simulink model "sim_BTMS"  (R2018b)
settings: Solver=FixedStepAuto  StartTime=0.0  StopTime=SimPara.t_sim  FixedStep=SimPara.t_step  RelTol=1e-3
values from neighbouring files (symbols this model uses):
  p = epe(jj).p    [main_sim_BTMS.m]    (also in main_sim_BTMS_1_system_setup.m = epe_mod(jj).p)
  SysPara = rmfield(SysPara, {'p','s'})    [main_sim_BTMS_1_system_setup.m]
undefined symbols (not defined in the file or in its folder): A, BatPara, BTMSConfig, i, LSAPara, SimPara, x2_cal, x3_cal, x_cal
libraries: simulink x14, dspstat3 x7, dspindex x1
(part 1 of 4)
Description:
  | A framework for the design and simulation of lithium-ion battery systems including the consideration of battery thermal management systems (BTMS).
  | Refer to https://github.com/TUMFTM/sim_BTMS for futher information.
  | 
  | Authors:
  | 
  | Christoph Reiter (christoph.reiter@tum.de)
  | Lars-Eric Schlereth
  | 
  | Created at:
  | 
  | Institute of Automotive Technology
  | Department of Mechanical Engineering
  | Technical University of Munich
settings Model: SimulationMode=accelerator  Creator=Christoph Reiter  LastModifiedBy=gu74niw
settings DataIOCC: SaveOutput=off  SignalLogging=off  DSMLogging=off  SaveTime=off  ReturnWorkspaceOutputs=on
settings OptimizationCC: SimCompilerOptimization=on

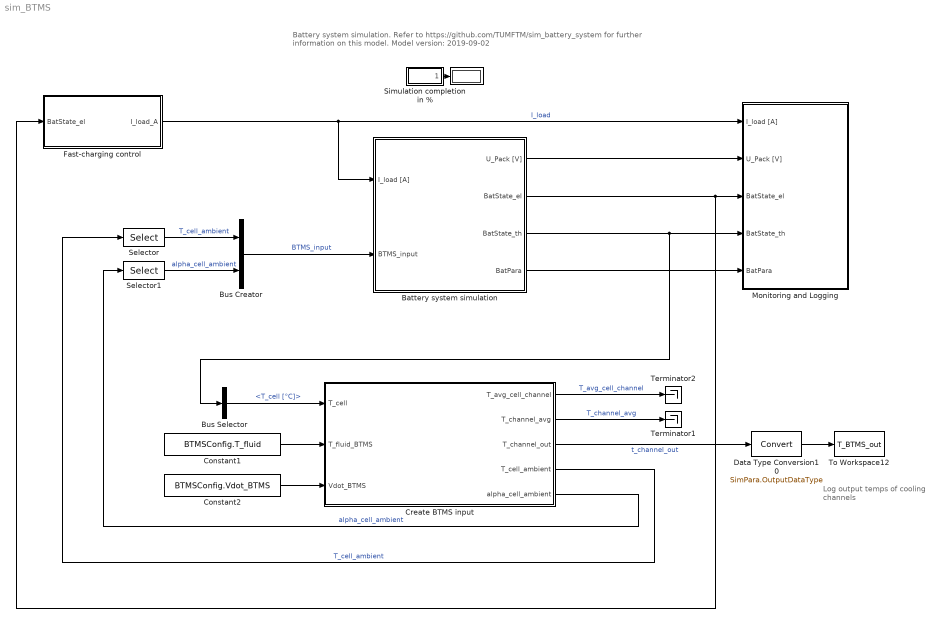
== system sim_BTMS ==
  note: Battery system simulation. Refer to https://github.com/TUMFTM/sim_battery_system for further information on this model.
      | Model version: 2019-09-02
  note: Log output temps of
      | cooling channels
  "\t\t      Simulation completion in %\t" : Subsystem
  " " : Display
      settings: Format=bank
  Battery system simulation : Subsystem  TreatAsAtomicUnit=on
  Bus Creator : BusCreator  Inputs=2
  Bus Selector : BusSelector  OutputSignals=T_cell [°C]
  Constant1 : Constant  Value=BTMSConfig.T_fluid
  Constant2 : Constant  Value=BTMSConfig.Vdot_BTMS
  Create BTMS input : Subsystem  Variant=on  VariantControl=Variant1
  Data Type Conversion10 : DataTypeConversion  OutDataTypeStr=SimPara.OutputDataType
  Fast-charging control : Subsystem
  Monitoring and Logging : Subsystem
  Selector : Selector  NumberOfDimensions=2  InputPortWidth=3  IndexOptions=Index vector (dialog),Index vector (dialog)  Indices=1:SysPara.p,1:SysPara.s  OutputSizes=1,1
  Selector1 : Selector  NumberOfDimensions=2  InputPortWidth=3  IndexOptions=Index vector (dialog),Index vector (dialog)  Indices=1:SysPara.p,1:SysPara.s  OutputSizes=1,1
  Terminator1 : Terminator
  Terminator2 : Terminator
  To Workspace12 : ToWorkspace  VariableName=T_BTMS_out  SaveFormat=Timeseries  SampleTime=-1
      settings: Decimation=SimPara.OutputDecimation
  wires:
  "\t\t      Simulation completion in %\t"/1(" ") -> " "/1
  Battery system simulation/1(U_Pack [V]) -> Monitoring and Logging/2(U_Pack [V])
  Battery system simulation/2(BatState_el) -> Fast-charging control/1(BatState_el), Monitoring and Logging/3(BatState_el)
  Battery system simulation/4(BatPara) -> Monitoring and Logging/5(BatPara)
  Battery system simulation/3(BatState_th) -> Bus Selector/1, Monitoring and Logging/4(BatState_th)
  Bus Creator/1 -> Battery system simulation/2(BTMS_input)  "BTMS_input"
  Bus Selector/1 -> Create BTMS input/1("T_cell ")  "<T_cell [°C]>"
  Constant1/1 -> Create BTMS input/2("T_fluid_BTMS ")
  Constant2/1 -> Create BTMS input/3("Vdot_BTMS ")
  Create BTMS input/1(" T_avg_cell_channel") -> Terminator2/1  "T_avg_cell_channel"
  Create BTMS input/3(" T_channel_out") -> Data Type Conversion10/1  "t_channel_out"
  Create BTMS input/4(" T_cell_ambient") -> Selector/1  "T_cell_ambient"
  Create BTMS input/5(" alpha_cell_ambient") -> Selector1/1  "alpha_cell_ambient"
  Create BTMS input/2(" T_channel_avg") -> Terminator1/1  "T_channel_avg"
  Fast-charging control/1(I_load_A) -> Battery system simulation/1(I_load [A]), Monitoring and Logging/1(I_load [A])  "I_load"
  Selector/1 -> Bus Creator/1  "T_cell_ambient"
  Selector1/1 -> Bus Creator/2  "alpha_cell_ambient"
  Data Type Conversion10/1 -> To Workspace12/1

== system sim_BTMS/		      Simulation completion in %	 ==
  note: Determine simulation completion
  Clock : Clock
  Divide : Product  Inputs=*/
  max. Simulaton Time : Constant  Value=SimPara.t_sim
  to % : Gain  Gain=100
  " " : Outport
  wires:
  max. Simulaton Time/1 -> Divide/2
  Clock/1 -> Divide/1
  Divide/1 -> to %/1
  to %/1 -> " "/1

== system sim_BTMS/Battery system simulation ==
  I_load [A] : Inport
  BTMS_input : Inport  Port=2
  Electrical Submodel : Subsystem
  Save BatState_el of last time-step : Subsystem
  Save BatState_th of last time-step : Subsystem
  Static and dynamic LIB parameters : Subsystem
  Thermal Submodel : Subsystem
  U_Pack [V] : Outport
  BatState_el : Outport  Port=2
  BatState_th : Outport  Port=3
  BatPara : Outport  Port=4
  wires:
  Static and dynamic LIB parameters/1(BatPara) -> Electrical Submodel/2(BatPara), Thermal Submodel/4(BatPara), BatPara/1
  Electrical Submodel/1(BatState_el) -> BatState_el/1, Save BatState_el of last time-step/1(BatState_el), Thermal Submodel/3(BatState_el)
  I_load [A]/1 -> Electrical Submodel/1(I_Pack [A])
  Electrical Submodel/2(U_Pack [V]) -> U_Pack [V]/1
  Save BatState_el of last time-step/1(BatState_el_in) -> Static and dynamic LIB parameters/2(BatState_el_in), Electrical Submodel/3(BatState_in)
  Thermal Submodel/1(BatState_th) -> BatState_th/1, Save BatState_th of last time-step/1(BatState_th)
  Save BatState_th of last time-step/1(Bat_State_th_in) -> Thermal Submodel/1(BatState_th_in), Static and dynamic LIB parameters/1(BatState_th_in)
  BTMS_input/1 -> Thermal Submodel/2(BTMS_input)

== system sim_BTMS/Create BTMS input ==
  "T_cell " : Inport
  "T_fluid_BTMS " : Inport  Port=2
  "Vdot_BTMS " : Inport  Port=3
  BTMS constant temp : Subsystem  VariantControl=SimPara.BTMS_sim_enable == 0
  BTMS fluid simulation : Subsystem  VariantControl=SimPara.BTMS_sim_enable == 1
  " T_avg_cell_channel" : Outport
  " T_channel_avg" : Outport  Port=2
  " T_channel_out" : Outport  Port=3
  " T_cell_ambient" : Outport  Port=4
  " alpha_cell_ambient" : Outport  Port=5

== system sim_BTMS/Fast-charging control ==
  note: Current reduction step
      | if max voltage is reached
  note: Detection of fully charged battery
  note: Overcharge-Protection
  BatState_el : Inport
  Add1 : Sum  Inputs=+-
  Battery fully charged : Constant  Value=SysPara.SOC_charge_max
  Bus Selector : BusSelector  OutputSignals=U_cell [V],SOC
  Constant1 : Constant  Value=SysPara.I_charge_min
  Constant2 : Constant
  Constant3 : Constant  Value=0
  Maximum : dspstat3/Maximum  operation=maximum  fcn=Value  indexBase=One  operateOver=Entire input  Dimension=1  InputProcessing=Columns as channels (frame based)  reset=None  roiEnable=off  roiType=Rectangles  roiPortion=Entire ROI  roiOutput=Individual statistics for each ROI  roiFlag=off  roundingMode=Floor  overflowMode=off  accumDataTypeStr=Inherit: Same as product output  accumLastDataTypeStr=Inherit: Same as product output
  Maximum1 : dspstat3/Maximum  operation=maximum  fcn=Value  indexBase=One  operateOver=Entire input  Dimension=1  InputProcessing=Columns as channels (frame based)  reset=None  roiEnable=off  roiType=Rectangles  roiPortion=Entire ROI  roiOutput=Individual statistics for each ROI  roiFlag=off  roundingMode=Floor  overflowMode=off  accumDataTypeStr=Inherit: Same as product output  accumLastDataTypeStr=Inherit: Same as product output
  Mean : dspstat3/Mean  run=off  InputProcessing=Columns as channels (frame based)  reset_popup=None  directionMode=Entire input  dimension=1  roiEnable=off  roiType=Rectangles  roiPortion=Entire ROI  roiOutput=Individual statistics for each ROI  roiFlag=off  roundingMode=Floor  overflowMode=off  outputDataTypeStr=Inherit: Same as accumulator  outputMin=[]  outputMax=[]  outputLastDataTypeStr=Inherit: Same as accumulator
  Relational Operator : RelationalOperator  OutDataTypeStr=boolean  RndMeth=Simplest
  Relational Operator2 : RelationalOperator  OutDataTypeStr=boolean  RndMeth=Simplest
  Stop Simulation : Stop
  Stop Simulation1 : Stop
  Switch1 : Switch  Threshold=SysPara.U_charge_target
  Unit Delay1 : UnitDelay  InitialCondition=SysPara.I_charge  SampleTime=-1
  Unit Delay2 : UnitDelay  InitialCondition=SysPara.I_charge  SampleTime=-1
  I_load_A : Outport
  wires:
  Unit Delay1/1 -> Add1/1
  Add1/1 -> Unit Delay1/1, Mean/1
  Relational Operator2/1 -> Stop Simulation1/1
  Switch1/1 -> Add1/2
  Constant1/1 -> Relational Operator2/1
  Constant2/1 -> Switch1/1
  Constant3/1 -> Switch1/3
  Bus Selector/1 -> Maximum/1  "<U_cell [V]>"
  Mean/1 -> Relational Operator2/2, Unit Delay2/1
  BatState_el/1 -> Bus Selector/1
  Maximum1/1 -> Relational Operator/1
  Battery fully charged/1 -> Relational Operator/2
  Relational Operator/1 -> Stop Simulation/1
  Bus Selector/2 -> Maximum1/1  "<SOC>"
  Maximum/1 -> Switch1/2
  Unit Delay2/1 -> I_load_A/1

== system sim_BTMS/Monitoring and Logging ==
  I_load [A] : Inport
  U_Pack [V] : Inport  Port=2
  BatState_el : Inport  Port=3
  BatState_th : Inport  Port=4
  BatPara : Inport  Port=5
  Constant : Constant  Value=SimPara.LoggingOutput
  Load Spectrum Analysis : Subsystem  Variant=on  VariantControl=Variant1
  Logging of Variables : Subsystem
  Temperature Sensor Simulation : Subsystem
  wires:
  I_load [A]/1 -> Logging of Variables/1(I_load [A])
  U_Pack [V]/1 -> Logging of Variables/2(U_Pack [A])
  BatState_el/1 -> Logging of Variables/3(BatState_el), Load Spectrum Analysis/1("BatState_el ")
  BatState_th/1 -> Temperature Sensor Simulation/1(bat_state_th_in)
  BatPara/1 -> Logging of Variables/5(BatPara), Load Spectrum Analysis/3("BatPara ")
  Constant/1 -> Logging of Variables/Enable
  Temperature Sensor Simulation/1(bat_state_th_out) -> Logging of Variables/4(BatState_th), Load Spectrum Analysis/2("BatState_th ")

== system sim_BTMS/Battery system simulation/Electrical Submodel ==
  note: Delay resulting balancing current for one step to avoid algebraic loop
  I_Pack [A] : Inport
  BatPara : Inport  Port=2
  BatState_in : Inport  Port=3
  Bus Creator1 : BusCreator  Inputs=8
  Cell Balancing : Subsystem
  Electric potential (single cell) : Subsystem
  Ohmic voltage drop and compensating currents in parallel connections : Subsystem
  Unit Delay4 : UnitDelay  InitialCondition=zeros(SysPara.p,SysPara.s)  SampleTime=-1
  Voltage of battery system : Subsystem
  dt : Subsystem
  BatState_el : Outport
  U_Pack [V] : Outport  Port=2
  wires:
  I_Pack [A]/1 -> Cell Balancing/1(I_Pack [A]), Ohmic voltage drop and compensating currents in parallel connections/2(I_Pack [A])
  Unit Delay4/1 -> Ohmic voltage drop and compensating currents in parallel connections/1(I_Balancing_in [A])  "I_Balancing_in [A]"
  Ohmic voltage drop and compensating currents in parallel connections/1(U_Cell [V]) -> Bus Creator1/1, Voltage of battery system/1(U_Cells [V]), Cell Balancing/2(U_Cell [V])
  Ohmic voltage drop and compensating currents in parallel connections/2(I_Cell [A]) -> Bus Creator1/2
  Ohmic voltage drop and compensating currents in parallel connections/3(U_R [V]) -> Bus Creator1/3
  Cell Balancing/1(I_Balancing [A]) -> Unit Delay4/1
  Voltage of battery system/1(U_Pack [V]) -> U_Pack [V]/1
  Bus Creator1/1 -> BatState_el/1  "BatState_el"
  BatPara/1 -> Ohmic voltage drop and compensating currents in parallel connections/3(BatPara), Electric potential (single cell)/1(BatPara)
  Electric potential (single cell)/1(U_Potential) -> Ohmic voltage drop and compensating currents in parallel connections/4(U_Potential [V]), Bus Creator1/4
  dt/1(dt [s]) -> Electric potential (single cell)/2(dt)
  BatState_in/1 -> Electric potential (single cell)/3(BatState_in)
  Electric potential (single cell)/2(SOC) -> Bus Creator1/5
  Electric potential (single cell)/3(U_OCV) -> Bus Creator1/6
  Electric potential (single cell)/4(U_Hysteresis) -> Bus Creator1/7
  Electric potential (single cell)/5(U_RC) -> Bus Creator1/8

== system sim_BTMS/Battery system simulation/Save BatState_el of last time-step ==
  note: Delay system state variables by one step to avoid algebraic loop.
      | We need these for the parameter lookup-tables
  BatState_el : Inport
  Bus Creator : BusCreator  Inputs=4
  Bus Creator2 : BusCreator  Inputs=4
  Bus Selector : BusSelector  OutputSignals=U_RC1 [V],U_RC2 [V],U_RC3 [V],U_RC4 [V]
  Bus Selector1 : BusSelector  OutputSignals=SOC,U_Hysteresis [V],I_cell [A],U_RC [V]
  Unit Delay : UnitDelay  InitialCondition=SysPara.BatStateInit.electrical.SOC  SampleTime=-1
  Unit Delay1 : UnitDelay  InitialCondition=SysPara.BatStateInit.electrical.U_hyst  SampleTime=-1
  Unit Delay2 : UnitDelay  InitialCondition=SysPara.BatStateInit.electrical.U_RC1  SampleTime=-1
  Unit Delay3 : UnitDelay  InitialCondition=SysPara.BatStateInit.electrical.U_RC2  SampleTime=-1
  Unit Delay4 : UnitDelay  InitialCondition=SysPara.BatStateInit.electrical.I_cell  SampleTime=-1
  Unit Delay5 : UnitDelay  InitialCondition=SysPara.BatStateInit.electrical.U_RC3  SampleTime=-1
  Unit Delay6 : UnitDelay  InitialCondition=SysPara.BatStateInit.electrical.U_RC4  SampleTime=-1
  BatState_el_in : Outport
  wires:
  Bus Selector1/2 -> Unit Delay1/1  "<U_Hysteresis [V]>"
  Unit Delay4/1 -> Bus Creator2/3  "I_cell [A]"
  Bus Selector1/3 -> Unit Delay4/1  "<I_cell [A]>"
  Unit Delay1/1 -> Bus Creator2/2  "U_Hysteresis [V]"
  Bus Selector1/1 -> Unit Delay/1  "<SOC>"
  Unit Delay/1 -> Bus Creator2/1  "SOC"
  Bus Creator2/1 -> BatState_el_in/1  "BatState_el_in"
  BatState_el/1 -> Bus Selector1/1
  Bus Selector1/4 -> Bus Selector/1  "<U_RC [V]>"
  Bus Selector/1 -> Unit Delay2/1  "<U_RC1 [V]>"
  Bus Selector/2 -> Unit Delay3/1  "<U_RC2 [V]>"
  Bus Selector/3 -> Unit Delay5/1  "<U_RC3 [V]>"
  Bus Selector/4 -> Unit Delay6/1  "<U_RC4 [V]>"
  Unit Delay6/1 -> Bus Creator/4  "U_RC4 [V]"
  Unit Delay5/1 -> Bus Creator/3  "U_RC3 [V]"
  Unit Delay3/1 -> Bus Creator/2  "U_RC2 [V]"
  Unit Delay2/1 -> Bus Creator/1  "U_RC1 [V]"
  Bus Creator/1 -> Bus Creator2/4  "U_RC"

== system sim_BTMS/Battery system simulation/Save BatState_th of last time-step ==
  note: Delay system state variables by one step to avoid algebraic loop.
      | We need these for the parameter lookup-tables
  BatState_th : Inport
  Bus Creator1 : BusCreator  Inputs=1
  Bus Selector : BusSelector  OutputSignals=T_cell [°C]
  Unit Delay1 : UnitDelay  InitialCondition=SysPara.BatStateInit.thermal.T_cell  SampleTime=-1
  Bat_State_th_in : Outport
  wires:
  Unit Delay1/1 -> Bus Creator1/1  "T_cell [°C]"
  Bus Selector/1 -> Unit Delay1/1  "<T_cell [°C]>"
  Bus Creator1/1 -> Bat_State_th_in/1  "Bat_State_th_in"
  BatState_th/1 -> Bus Selector/1

== system sim_BTMS/Battery system simulation/Static and dynamic LIB parameters ==
  BatState_th_in : Inport
  BatState_el_in : Inport  Port=2
  LIB Parameter Look-Ups : Subsystem
  Statistic Cell Deviations : Subsystem
  BatPara : Outport
  wires:
  LIB Parameter Look-Ups/1(BatPara_el_uniform) -> Statistic Cell Deviations/1("BatPara_el_uniform ")
  Statistic Cell Deviations/1(BatPara) -> BatPara/1  "BatPara"
  BatState_el_in/1 -> LIB Parameter Look-Ups/2(BatState_el_in)
  BatState_th_in/1 -> LIB Parameter Look-Ups/1(BatState_th_in)

== system sim_BTMS/Battery system simulation/Thermal Submodel ==
  note: Total cell heat generation:
      |
      | PQ_cell = PQ_cell,irr + PQ_cell,rev
  BatState_th_in : Inport
  BTMS_input : Inport  Port=2
  BatState_el : Inport  Port=3
  BatPara : Inport  Port=4
  Add : Sum
  Bus Creator : BusCreator  Inputs=6
  Bus Selector : BusSelector  OutputSignals=U_R [V],U_RC [V],I_cell [A]
  Bus Selector3 : BusSelector  OutputSignals=alpha_cell_ambient,T_cell_ambient
  Bus Selector4 : BusSelector  OutputSignals=T_cell [°C]
  Cell heat transport and heat dissipation : Subsystem
  Constant : Constant  Value=SimPara.thermal_sim_enable
  Irreversible heat generation : Subsystem
  Reversible heat generation : Subsystem
  BatState_th : Outport
  wires:
  Bus Selector3/2 -> Cell heat transport and heat dissipation/5(T_cell_ambient), Bus Creator/5  "<T_cell_ambient>"
  Add/1 -> Cell heat transport and heat dissipation/1(PQ_cell), Bus Creator/1  "PQ_cell [W]"
  Bus Creator/1 -> BatState_th/1  "BatState_th"
  Bus Selector3/1 -> Cell heat transport and heat dissipation/4(alpha_cell_ambient), Bus Creator/6  "<alpha_cell_ambient>"
  Irreversible heat generation/1(PQ_cell,irr [W]) -> Add/1
  Reversible heat generation/1(PQ_cell,rev [W]) -> Add/2
  BatPara/1 -> Cell heat transport and heat dissipation/2(BatPara), Reversible heat generation/3(BatPara)
  BatState_el/1 -> Bus Selector/1
  Bus Selector/2 -> Irreversible heat generation/2(U_RC)  "<U_RC [V]>"
  Bus Selector/3 -> Reversible heat generation/1(I_Cells [A]), Irreversible heat generation/3(I_Cells [A])  "<I_cell [A]>"
  Bus Selector/1 -> Irreversible heat generation/1(U_R [V])  "<U_R [V]>"
  BTMS_input/1 -> Bus Selector3/1
  BatState_th_in/1 -> Bus Selector4/1
  Bus Selector4/1 -> Reversible heat generation/2(T_Cells [°C]), Cell heat transport and heat dissipation/3(T_cell_in)  "<T_cell [°C]>"
  Cell heat transport and heat dissipation/1(T_cell [°C]) -> Bus Creator/2
  Constant/1 -> Cell heat transport and heat dissipation/Enable
  Cell heat transport and heat dissipation/3(PQ_transfer [W]) -> Bus Creator/4
  Cell heat transport and heat dissipation/2(PQ_ambient [W]) -> Bus Creator/3

== system sim_BTMS/Create BTMS input/BTMS constant temp ==
  note: BTMS simulation switched off, assuming constand ambient cell temperatures and heat transfer coefficients.
  "T_cell " : Inport
  "T_fluid_BTMS " : Inport  Port=2
  "Vdot_BTMS " : Inport  Port=3
  Constant : Constant  Value=SysPara.thermal.T_cell_ambient*ones(SysPara.p, SysPara.s)
  Constant3 : Constant  Value=SysPara.thermal.alpha_cell_ambient*ones(SysPara.p, SysPara.s)
  Ground : Ground
  Ground1 : Ground
  Ground2 : Ground
  Terminator : Terminator
  Terminator1 : Terminator
  Terminator2 : Terminator
  " T_avg_cell_channel" : Outport
  " T_channel_avg" : Outport  Port=2
  " T_channel_out" : Outport  Port=3
  " T_cell_ambient" : Outport  Port=4
  " alpha_cell_ambient" : Outport  Port=5
  wires:
  "T_cell "/1 -> Terminator/1
  "T_fluid_BTMS "/1 -> Terminator1/1
  "Vdot_BTMS "/1 -> Terminator2/1
  Ground1/1 -> " T_channel_avg"/1
  Constant/1 -> " T_cell_ambient"/1  "T_cell_ambient"
  Constant3/1 -> " alpha_cell_ambient"/1  "alpha_cell_ambient"
  Ground2/1 -> " T_channel_out"/1
  Ground/1 -> " T_avg_cell_channel"/1

== system sim_BTMS/Create BTMS input/BTMS fluid simulation ==
  note: Use T_cell of last time-step
      | to avoid algebraic loop
  "T_cell " : Inport
  "T_fluid_BTMS " : Inport  Port=2
  "Vdot_BTMS " : Inport  Port=3
  BTMS fluid simulation function : MATLAB Function  TreatAsAtomicUnit=on  VariantControl=Variant1
  Constant1 : Constant  Value=SysPara.thermal.transfer.A_y
  Constant2 : Constant  Value=SysPara.thermal.transfer.A_z
  Constant3 : Constant  Value=SysPara.thermal.transfer.A_x
  Constant4 : Constant  Value=SysPara.s
  Constant5 : Constant  Value=SysPara.p
  Unit Delay : UnitDelay  InitialCondition=SysPara.BatStateInit.electrical.SOC  SampleTime=-1
  " T_avg_cell_channel" : Outport
  " T_channel_avg" : Outport  Port=2
  " T_channel_out" : Outport  Port=3
  " T_cell_ambient" : Outport  Port=4
  " alpha_cell_ambient" : Outport  Port=5
  wires:
  "T_cell "/1 -> Unit Delay/1
  "T_fluid_BTMS "/1 -> BTMS fluid simulation function/2(T_fluid_BTMS)
  "Vdot_BTMS "/1 -> BTMS fluid simulation function/3(Vdot_BTMS)
  BTMS fluid simulation function/1(T_avg_cell_channel) -> " T_avg_cell_channel"/1
  BTMS fluid simulation function/2(T_channel_avg) -> " T_channel_avg"/1
  BTMS fluid simulation function/3(T_channel_out) -> " T_channel_out"/1
  BTMS fluid simulation function/4(T_cell_ambient) -> " T_cell_ambient"/1
  BTMS fluid simulation function/5(alpha_cell_ambient) -> " alpha_cell_ambient"/1
  Constant3/1 -> BTMS fluid simulation function/4(A_x)  "alpha_cell_ambient"
  Constant1/1 -> BTMS fluid simulation function/5(A_y)  "alpha_cell_ambient"
  Constant2/1 -> BTMS fluid simulation function/6(A_z)  "alpha_cell_ambient"
  Constant4/1 -> BTMS fluid simulation function/7(s)  "alpha_cell_ambient"
  Constant5/1 -> BTMS fluid simulation function/8(p)  "alpha_cell_ambient"
  Unit Delay/1 -> BTMS fluid simulation function/1(T_cell)  "T_cell"

== system sim_BTMS/Monitoring and Logging/Load Spectrum Analysis ==
  "BatState_el " : Inport
  "BatState_th " : Inport  Port=2
  "BatPara " : Inport  Port=3
  Load Spectrum Analysis OFF : Subsystem  VariantControl=SimPara.LoadSpectra_enable == 0
  Load Spectrum Analysis ON : Subsystem  VariantControl=SimPara.LoadSpectra_enable == 1

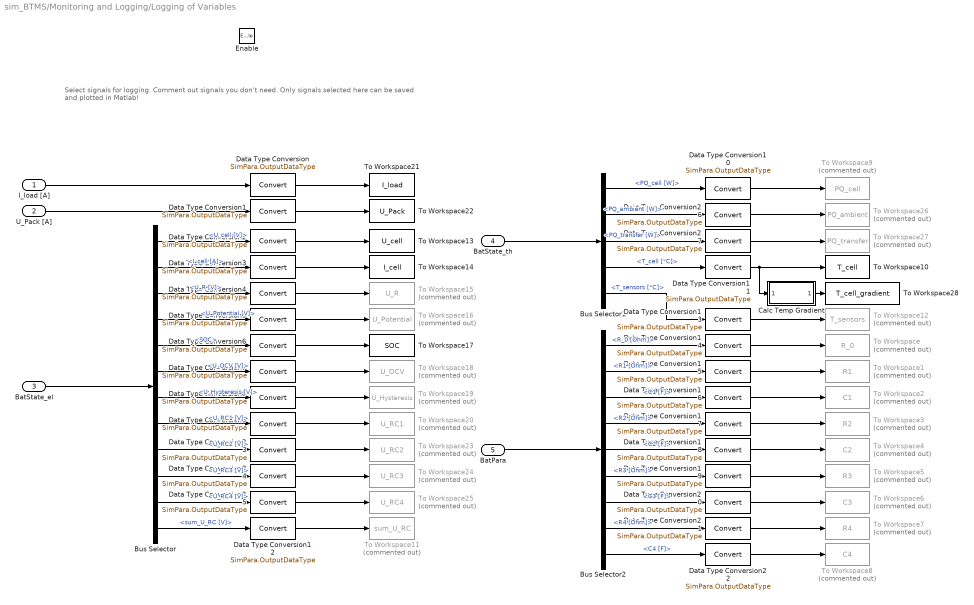
== system sim_BTMS/Monitoring and Logging/Logging of Variables ==
  note: Select signals for logging. Comment out signals you don't need.
      | Only signals selected here can be saved and plotted in Matlab!
  I_load [A] : Inport
  U_Pack [A] : Inport  Port=2
  BatState_el : Inport  Port=3
  BatState_th : Inport  Port=4
  BatPara : Inport  Port=5
  Enable : EnablePort
  Bus Selector : BusSelector  OutputSignals=U_cell [V],I_cell [A],U_R [V],U_Potential [V],SOC,U_OCV [V],U_Hysteresis [V],U_RC [V].U_RC1 [V],U_RC [V].U_RC2 [V],U_RC [V].U_RC3 [V],U_RC [V].U_RC4 [V],U_RC [V].sum_U_RC [V]
  Bus Selector1 : BusSelector  OutputSignals=PQ_cell [W],PQ_ambient [W],PQ_transfer [W],T_cell [°C],T_sensors [°C]
  Bus Selector2 : BusSelector  OutputSignals=electrical.R_0 [Ohm],electrical.R1 [Ohm],electrical.C1 [F],electrical.R2 [Ohm],electrical.C2 [F],electrical.R3 [Ohm],electrical.C3 [F],electrical.R4 [Ohm],electrical.C4 [F]
  Calc Temp Gradient : Subsystem
  Data Type Conversion{,1..27} (28 alike) : DataTypeConversion  OutDataTypeStr=SimPara.OutputDataType
  To Workspace : ToWorkspace  Commented=on  VariableName=R_0  SaveFormat=Timeseries  SampleTime=-1
      settings: Decimation=SimPara.OutputDecimation
  To Workspace1 : ToWorkspace  Commented=on  VariableName=R1  SaveFormat=Timeseries  SampleTime=-1
      settings: Decimation=SimPara.OutputDecimation
  To Workspace10 : ToWorkspace  VariableName=T_cell  SaveFormat=Timeseries  SampleTime=-1
      settings: Decimation=SimPara.OutputDecimation
  To Workspace11 : ToWorkspace  Commented=on  VariableName=sum_U_RC  SaveFormat=Timeseries  SampleTime=-1
      settings: Decimation=SimPara.OutputDecimation
  To Workspace12 : ToWorkspace  Commented=on  VariableName=T_sensors  SaveFormat=Timeseries  SampleTime=-1
      settings: Decimation=SimPara.OutputDecimation
  To Workspace13 : ToWorkspace  VariableName=U_cell  SaveFormat=Timeseries  SampleTime=-1
      settings: Decimation=SimPara.OutputDecimation
  To Workspace14 : ToWorkspace  VariableName=I_cell  SaveFormat=Timeseries  SampleTime=-1
      settings: Decimation=SimPara.OutputDecimation
  To Workspace15 : ToWorkspace  Commented=on  VariableName=U_R  SaveFormat=Timeseries  SampleTime=-1
      settings: Decimation=SimPara.OutputDecimation
  To Workspace16 : ToWorkspace  Commented=on  VariableName=U_Potential  SaveFormat=Timeseries  SampleTime=-1
      settings: Decimation=SimPara.OutputDecimation
  To Workspace17 : ToWorkspace  VariableName=SOC  SaveFormat=Timeseries  SampleTime=-1
      settings: Decimation=SimPara.OutputDecimation
  To Workspace18 : ToWorkspace  Commented=on  VariableName=U_OCV  SaveFormat=Timeseries  SampleTime=-1
      settings: Decimation=SimPara.OutputDecimation
  To Workspace19 : ToWorkspace  Commented=on  VariableName=U_Hysteresis  SaveFormat=Timeseries  SampleTime=-1
      settings: Decimation=SimPara.OutputDecimation
  To Workspace2 : ToWorkspace  Commented=on  VariableName=C1  SaveFormat=Timeseries  SampleTime=-1
      settings: Decimation=SimPara.OutputDecimation
  To Workspace20 : ToWorkspace  Commented=on  VariableName=U_RC1  SaveFormat=Timeseries  SampleTime=-1
      settings: Decimation=SimPara.OutputDecimation
  To Workspace21 : ToWorkspace  VariableName=I_load  SaveFormat=Timeseries  SampleTime=-1
      settings: Decimation=SimPara.OutputDecimation
  To Workspace22 : ToWorkspace  VariableName=U_Pack  SaveFormat=Timeseries  SampleTime=-1
      settings: Decimation=SimPara.OutputDecimation
  To Workspace23 : ToWorkspace  Commented=on  VariableName=U_RC2  SaveFormat=Timeseries  SampleTime=-1
      settings: Decimation=SimPara.OutputDecimation
  To Workspace24 : ToWorkspace  Commented=on  VariableName=U_RC3  SaveFormat=Timeseries  SampleTime=-1
      settings: Decimation=SimPara.OutputDecimation
  To Workspace25 : ToWorkspace  Commented=on  VariableName=U_RC4  SaveFormat=Timeseries  SampleTime=-1
      settings: Decimation=SimPara.OutputDecimation
  To Workspace26 : ToWorkspace  Commented=on  VariableName=PQ_ambient  SaveFormat=Timeseries  SampleTime=-1
      settings: Decimation=SimPara.OutputDecimation
  To Workspace27 : ToWorkspace  Commented=on  VariableName=PQ_transfer  SaveFormat=Timeseries  SampleTime=-1
      settings: Decimation=SimPara.OutputDecimation
  To Workspace28 : ToWorkspace  VariableName=T_cell_gradient  SaveFormat=Timeseries  SampleTime=-1
      settings: Decimation=SimPara.OutputDecimation
  To Workspace3 : ToWorkspace  Commented=on  VariableName=R2  SaveFormat=Timeseries  SampleTime=-1
      settings: Decimation=SimPara.OutputDecimation
  To Workspace4 : ToWorkspace  Commented=on  VariableName=C2  SaveFormat=Timeseries  SampleTime=-1
      settings: Decimation=SimPara.OutputDecimation
  To Workspace5 : ToWorkspace  Commented=on  VariableName=R3  SaveFormat=Timeseries  SampleTime=-1
      settings: Decimation=SimPara.OutputDecimation
  To Workspace6 : ToWorkspace  Commented=on  VariableName=C3  SaveFormat=Timeseries  SampleTime=-1
      settings: Decimation=SimPara.OutputDecimation
  To Workspace7 : ToWorkspace  Commented=on  VariableName=R4  SaveFormat=Timeseries  SampleTime=-1
      settings: Decimation=SimPara.OutputDecimation
  To Workspace8 : ToWorkspace  Commented=on  VariableName=C4  SaveFormat=Timeseries  SampleTime=-1
      settings: Decimation=SimPara.OutputDecimation
  To Workspace9 : ToWorkspace  Commented=on  VariableName=PQ_cell  SaveFormat=Timeseries  SampleTime=-1
      settings: Decimation=SimPara.OutputDecimation
  wires:
  Data Type Conversion2/1 -> To Workspace13/1
  Bus Selector2/3 -> Data Type Conversion16/1  "<C1 [F]>"
  Data Type Conversion6/1 -> To Workspace17/1
  Bus Selector2/4 -> Data Type Conversion17/1  "<R2 [Ohm]>"
  Data Type Conversion8/1 -> To Workspace19/1
  Bus Selector1/4 -> Data Type Conversion11/1  "<T_cell [°C]>"
  Data Type Conversion14/1 -> To Workspace/1
  Bus Selector1/1 -> Data Type Conversion10/1  "<PQ_cell [W]>"
  U_Pack [A]/1 -> Data Type Conversion1/1
  Bus Selector/11 -> Data Type Conversion25/1  "<U_RC4 [V]>"
  Bus Selector2/7 -> Data Type Conversion20/1  "<C3 [F]>"
  Bus Selector/5 -> Data Type Conversion6/1  "<SOC>"
  Bus Selector/10 -> Data Type Conversion24/1  "<U_RC3 [V]>"
  Bus Selector2/6 -> Data Type Conversion19/1  "<R3 [Ohm]>"
  Bus Selector2/2 -> Data Type Conversion15/1  "<R1 [Ohm]>"
  Bus Selector/12 -> Data Type Conversion12/1  "<sum_U_RC [V]>"
  Bus Selector/3 -> Data Type Conversion4/1  "<U_R [V]>"
  Bus Selector/7 -> Data Type Conversion8/1  "<U_Hysteresis [V]>"
  BatPara/1 -> Bus Selector2/1
  Bus Selector2/5 -> Data Type Conversion18/1  "<C2 [F]>"
  Data Type Conversion23/1 -> To Workspace23/1
  Data Type Conversion/1 -> To Workspace21/1
  Bus Selector2/9 -> Data Type Conversion22/1  "<C4 [F]>"
  Bus Selector/2 -> Data Type Conversion3/1  "<I_cell [A]>"
  Bus Selector/1 -> Data Type Conversion2/1  "<U_cell [V]>"
  Bus Selector/6 -> Data Type Conversion7/1  "<U_OCV [V]>"
  Data Type Conversion17/1 -> To Workspace3/1
  Data Type Conversion24/1 -> To Workspace24/1
  Data Type Conversion3/1 -> To Workspace14/1
  Data Type Conversion5/1 -> To Workspace16/1
  Data Type Conversion9/1 -> To Workspace20/1
  Data Type Conversion4/1 -> To Workspace15/1
  Data Type Conversion15/1 -> To Workspace1/1
  Data Type Conversion11/1 -> To Workspace10/1, Calc Temp Gradient/1(T_cell)
  Data Type Conversion22/1 -> To Workspace8/1
  Data Type Conversion20/1 -> To Workspace6/1
  Data Type Conversion19/1 -> To Workspace5/1
  Data Type Conversion10/1 -> To Workspace9/1
  Data Type Conversion16/1 -> To Workspace2/1
  Data Type Conversion1/1 -> To Workspace22/1
  Data Type Conversion7/1 -> To Workspace18/1
  Bus Selector2/1 -> Data Type Conversion14/1  "<R_0 [Ohm]>"
  Data Type Conversion25/1 -> To Workspace25/1
  Bus Selector/8 -> Data Type Conversion9/1  "<U_RC1 [V]>"
  Data Type Conversion18/1 -> To Workspace4/1
  Data Type Conversion12/1 -> To Workspace11/1
  Bus Selector/4 -> Data Type Conversion5/1  "<U_Potential [V]>"
  Bus Selector/9 -> Data Type Conversion23/1  "<U_RC2 [V]>"
  Data Type Conversion21/1 -> To Workspace7/1
  I_load [A]/1 -> Data Type Conversion/1
  BatState_el/1 -> Bus Selector/1
  Bus Selector2/8 -> Data Type Conversion21/1  "<R4 [Ohm]>"
  BatState_th/1 -> Bus Selector1/1
  Data Type Conversion13/1 -> To Workspace12/1
  Bus Selector1/5 -> Data Type Conversion13/1  "<T_sensors [°C]>"
  Data Type Conversion27/1 -> To Workspace27/1
  Data Type Conversion26/1 -> To Workspace26/1
  Bus Selector1/2 -> Data Type Conversion26/1  "<PQ_ambient [W]>"
  Bus Selector1/3 -> Data Type Conversion27/1  "<PQ_transfer [W]>"
  Calc Temp Gradient/1(T_cell_gradient) -> To Workspace28/1

== system sim_BTMS/Monitoring and Logging/Temperature Sensor Simulation ==
  bat_state_th_in : Inport
  Bus Selector : BusSelector  OutputSignals=T_cell [°C]
  Enable/disable temperature sensors : Subsystem  Variant=on
  Rebuild bus structure : Subsystem
  bat_state_th_out : Outport
  wires:
  bat_state_th_in/1 -> Bus Selector/1, Rebuild bus structure/2(Bat_state_th_in)
  Bus Selector/1 -> Enable/disable temperature sensors/1(T_cell)  "<T_cell [°C]>"
  Enable/disable temperature sensors/1(T_sensors [°C]) -> Rebuild bus structure/1(T_sensors)
  Rebuild bus structure/1(bat_state_th_out) -> bat_state_th_out/1

== system sim_BTMS/Battery system simulation/Electrical Submodel/Cell Balancing ==
  note: The balancing function is only active if the following three conditions are met:
  note: -> Da zu einem Auswertungszeitpunkt das Stattfinden von Balancing auf Basis der Klemmenspannungen der Zellen bestimmt wird und die Balancing-Ströme der Zellen ebenfalls über deren Klemmenspannungen berechnet werden, können bei Balancing-Auftritt diese Balancing-Ströme erst zum nächsten Auswertungszeitpunkt für die Berechnung der neuen Klemmenspannungen und Strombelastungen der Zellen verwendet werden
      | -> Dadurch wird ein Fehler gemacht, der im diskreten Modell jedoch unvermeidbar ist
  note: Simple dissipative balancing.
      | Attention: For maximum flexibility of the model it is assumed every cell has it's own balancing resistor. Of course, in a parallel connection the equalisation effects allow the cells to share one balancing resistor. Therefore, a parallel connection of 5 cells with a balancing resistor of 33 Ohm would be set up like this: SysPara.Balancing.R = 33/5
  note: Condition 1: Terminal voltages of all cells in the battery pack >= Balancing.U_Limit
  note: The lowest terminal voltage of all cells in the battery pack always serves as reference.
      | à If the voltage difference between the terminal voltage of a cell and the reference voltage is greater than Balancing.U_Delta, this cell is connected to its balancing resistor.
      | à Condition for balancing: U_cell - reference voltage > Balancing.U_Delta
      | à It is not enough, if the voltage difference is equal to Balancing.U_Delta à The reason for this is that otherwise, with Balancing.U_Delta = 0, the cells with the lowest terminal voltage would also have their balancing resistors switched on.
  note: Determination of the balancing currents of the cells:
      | à The balancing current is the current that loads the cell when the balancing resistor is switched on.
      | à Calculation via the terminal voltages of the cells and via the balancing resistances of the cells using Ohm's law
      | à A negative sign must be considered in the equation because the balancing current discharges a cell and currents are defined negatively in the battery pack model for discharging.
      | I_Balancing = - U_cell / Balancing.R
  note: Condition 2: Amount of the external current load of the battery pack <= Balancing.I_Limit
  note: Condition 3: Simulation time >= Balancing.t_Start
  I_Pack [A] : Inport
  U_Cell [V] : Inport  Port=2
  Abs : Abs
  Clock : Clock
  Constant : Constant  Value=SysPara.Balancing.R  VectorParams1D=off
  Constant1 : Constant  Value=SysPara.Balancing.U_Delta  VectorParams1D=off
  Constant2 : Constant  Value=SysPara.Balancing.U_Limit  VectorParams1D=off
  Constant3 : Constant  Value=SysPara.Balancing.I_Limit  VectorParams1D=off
  Constant4 : Constant  Value=SysPara.Balancing.t_Start
  Divide : Product  Inputs=/*
  Gain : Gain  Gain=-1  OutDataTypeStr=double
  Minimum : dspstat3/Minimum  operation=minimum  fcn=Value  indexBase=One  operateOver=Entire input  Dimension=1  InputProcessing=Columns as channels (frame based)  reset=None  roiEnable=off  roiType=Rectangles  roiPortion=Entire ROI  roiOutput=Individual statistics for each ROI  roiFlag=off  roundingMode=Floor  overflowMode=off
      settings: SourceProductName=DSP System Toolbox  SourceProductBaseCode=DS
  Product : Product  Inputs=5
  Relational Operator : RelationalOperator  Operator=>  OutDataTypeStr=boolean  RndMeth=Simplest
  Relational Operator1 : RelationalOperator  OutDataTypeStr=boolean  RndMeth=Simplest
  Relational Operator2 : RelationalOperator  Operator=<=  OutDataTypeStr=boolean  RndMeth=Simplest
  Relational Operator3 : RelationalOperator  OutDataTypeStr=boolean  RndMeth=Simplest
  Subtract : Sum  Inputs=+-
  I_Balancing [A] : Outport
  wires:
  U_Cell [V]/1 -> Minimum/1, Divide/2, Subtract/1
  Product/1 -> I_Balancing [A]/1  "I_Balancing [A]"
  Minimum/1 -> Relational Operator1/1, Subtract/2
  Constant/1 -> Divide/1
  Constant1/1 -> Relational Operator/2
  I_Pack [A]/1 -> Abs/1
  Constant3/1 -> Relational Operator2/2
  Clock/1 -> Relational Operator3/1
  Constant4/1 -> Relational Operator3/2
  Constant2/1 -> Relational Operator1/2
  Relational Operator3/1 -> Product/5
  Relational Operator2/1 -> Product/4
  Relational Operator1/1 -> Product/3
  Relational Operator/1 -> Product/2
  Divide/1 -> Gain/1
  Gain/1 -> Product/1
  Abs/1 -> Relational Operator2/1
  Subtract/1 -> Relational Operator/1

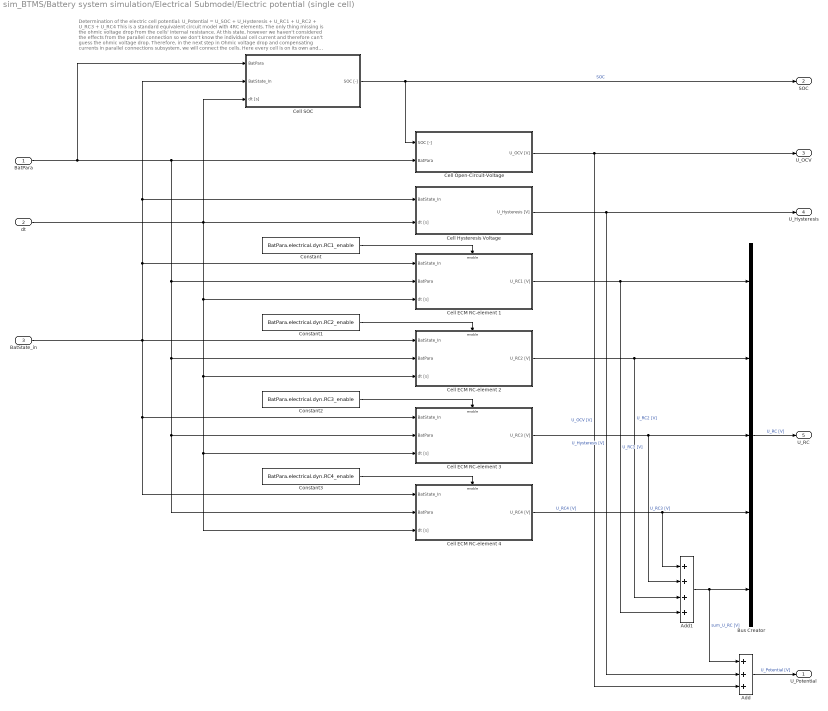
== system sim_BTMS/Battery system simulation/Electrical Submodel/Electric potential (single cell) ==
  note: Determination of the electric cell potential: U_Potential = U_SOC + U_Hysteresis + U_RC1 + U_RC2 + U_RC3 + U_RC4
      |
      | This is a standard equivalent circuit model with 4RC elements. The only thing missing is the ohmic voltage drop from the cells' internal resistance. At this state, however we haven't considered the effects from the parallel connection so we don't know the individual cell current and therefore can't guess the ohmic voltage drop. Therefore, in the next step in Ohmic voltage drop and compensating currents in parallel connections subsystem, we will connect the cells. Here every cell is on its own and doesn't interact with the other cells ins the syster (yet).
  BatPara : Inport
  dt : Inport  Port=2
  BatState_in : Inport  Port=3
  Add : Sum  Inputs=+++
  Add1 : Sum  Inputs=++++
  Bus Creator : BusCreator  Inputs=5
  Cell ECM RC-element 1 : Subsystem
  Cell ECM RC-element 2 : Subsystem
  Cell ECM RC-element 3 : Subsystem
  Cell ECM RC-element 4 : Subsystem
  Cell Hysteresis Voltage : Subsystem
  Cell Open-Circuit-Voltage : Subsystem
  Cell SOC : Subsystem
  Constant : Constant  Value=BatPara.electrical.dyn.RC1_enable
  Constant1 : Constant  Value=BatPara.electrical.dyn.RC2_enable
  Constant2 : Constant  Value=BatPara.electrical.dyn.RC3_enable
  Constant3 : Constant  Value=BatPara.electrical.dyn.RC4_enable
  U_Potential : Outport
  SOC : Outport  Port=2
  U_OCV : Outport  Port=3
  U_Hysteresis : Outport  Port=4
  U_RC : Outport  Port=5
  wires:
  BatState_in/1 -> Cell ECM RC-element 4/1(BatState_In), Cell ECM RC-element 3/1(BatState_In), Cell ECM RC-element 2/1(BatState_In), Cell Hysteresis Voltage/1(BatState_In), Cell SOC/2(BatState_In), Cell ECM RC-element 1/1(BatState_In)
  Cell ECM RC-element 1/1(U_RC1 [V]) -> Add1/4, Bus Creator/1  "U_RC1 [V]"
  Cell SOC/1(SOC [-]) -> Cell Open-Circuit-Voltage/1(SOC [-]), SOC/1  "SOC"
  Cell Open-Circuit-Voltage/1(U_OCV [V]) -> Add/3, U_OCV/1  "U_OCV [V]"
  dt/1 -> Cell ECM RC-element 4/3(dt [s]), Cell ECM RC-element 3/3(dt [s]), Cell ECM RC-element 2/3(dt [s]), Cell ECM RC-element 1/3(dt [s]), Cell SOC/3(dt [s]), Cell Hysteresis Voltage/2(dt [s])
  Cell ECM RC-element 2/1(U_RC2 [V]) -> Add1/3, Bus Creator/2  "U_RC2 [V]"
  BatPara/1 -> Cell Open-Circuit-Voltage/2(BatPara), Cell ECM RC-element 1/2(BatPara), Cell ECM RC-element 2/2(BatPara), Cell ECM RC-element 3/2(BatPara), Cell ECM RC-element 4/2(BatPara), Cell SOC/1(BatPara)
  Cell Hysteresis Voltage/1(U_Hysteresis [V]) -> Add/2, U_Hysteresis/1  "U_Hysteresis [V]"
  Add/1 -> U_Potential/1  "U_Potential [V]"
  Cell ECM RC-element 3/1(U_RC3 [V]) -> Add1/2, Bus Creator/3  "U_RC3 [V]"
  Cell ECM RC-element 4/1(U_RC4 [V]) -> Add1/1, Bus Creator/4  "U_RC4 [V]"
  Bus Creator/1 -> U_RC/1  "U_RC [V]"
  Add1/1 -> Add/1, Bus Creator/5  "sum_U_RC [V]"
  Constant/1 -> Cell ECM RC-element 1/Enable
  Constant1/1 -> Cell ECM RC-element 2/Enable
  Constant2/1 -> Cell ECM RC-element 3/Enable
  Constant3/1 -> Cell ECM RC-element 4/Enable

== system sim_BTMS/Battery system simulation/Electrical Submodel/Ohmic voltage drop and compensating currents in parallel connections ==
  note: Now it gets complicated… In this step the cells are connected in serial and parallel and the current distribution in the parallel connection as well as the compensating currents are calculated. The calculation makes heavy use of the matrix structure of the signals so many things happen at ones. Here follows a shot summary of what happens here.
      | Steps for determining the terminal voltages and current loads of the cells:
      | 1. Assumption of the interconnection mechanism of the cells: Cells are first connected in parallel to a network -> parallel cell networks are then connected in series
      | 2. Determination of the current loads of the cells connected in parallel, which consider the compensating currents, by means of a backward calculation using the terminal voltages of the cells and knowledge of the potentials and ohmic internal resistances of the cells.
      | 3. Terminal voltages of the cells in a parallel cell system = terminal voltage of the parallel cell system
      | 4. Calculation of the terminal voltage of a parallel cell system via a representative total current in the parallel cell system and via a substitute resistance of the parallel cell system using Ohm's law.
      | 5. For the representative total current in a parallel cell network, the information about the potentials of the cells in this network must be considered à This is possible via the short-circuit currents of the cells in this network.
      | 6. The further proportions of the representative total current in a parallel cell system refer to an occurring current load -> External current load of the battery pack, because this is present at each parallel cell system due to the assumed interconnection mechanism in the battery pack model, and balancing currents of the cells in this system.
      | 7. The equivalent resistance of a parallel cell composite results from the total resistances of the individual cells in this composite.
      |
      | Determination of the terminal voltages of the cells:
      | 1. short-circuit currents of the cells = U_Potential / R_0 (ohmic internal resistances of the cells)
      | è Short circuit current of a cell contains the information about the potential of the cell.
      | è Calculation background: The electrical equivalent circuit of a cell is simplified to the potential of the cell and the ohmic internal resistance of the cell à When the cell is short-circuited, the entire potential of the cell drops at the ohmic internal resistance of the cell.
      | 2. Addition of the short-circuit currents of the cells via cells connected in parallel
      | 3. Add I_load (external current load of the battery pack) to each parallel cell array.
      | 4. Adding of I_Balancing (see subsystem "Balancing") to the cells via parallel connected cells
      | 5. The sum of these currents gives the representative total current in each parallel cell system or the total current in each parallel cell system including consideration of the short circuits of the cells.
      | 6. For the simplified equivalent electrical circuit, which is used for the realization of the equalizing currents, the total resistance of a cell consists only of the ohmic internal resistance of the cell
      | è Determination of the equivalent resistance of a parallel cell network via parallel connection of the ohmic internal resistances of the cells in this network
      | è Add up the reciprocal values of the ohmic internal resistances of the cells via cells connected in parallel: 1/R_ges = 1/R_1 + 1/R_2 + ...
      | è Replacement resistance of a parallel cell network corresponds to the reciprocal value of the result
      | 7. Terminal voltage of a parallel cell system = total current in the parallel cell system including consideration of the short circuits of the cells * Replacement resistance of the parallel cell system = terminal voltage of each cell in the parallel cell system because cells connected in parallel have the same terminal voltage
      | è U_cell (terminal voltages of the cells) successfully calculated
      |
      | Determination of the current loads of the cells:
      | 1. U_R (ohmic voltage components of the cells) = U_cell - U_Potential
      | 2. I_cell (current loads of the cells) = U_R / R_0
      |
      | Result:
      | à I_cell considers the equalizing currents in a parallel cell array, which always ensure identical terminal voltages of the cells in this array -> Physical condition in a parallel cell array
      | à The short-circuit currents of the cells are included in the calculation so that the potentials of the cells can be considered when calculating the terminal voltage.
      | à For U_R = U_cell - U_Potential the potentials of the individual cells are calculated again.
      | à Sum of the current loads of the cells in a parallel cell network = External current load of the battery pack + Sum of the balancing currents of the cells in this network -> Correct physical correlation
  I_Balancing_in [A] : Inport
  I_Pack [A] : Inport  Port=2
  BatPara : Inport  Port=3
  U_Potential [V] : Inport  Port=4
  Add : Sum  Inputs=+++
  Bus Selector1 : BusSelector  OutputSignals=electrical.R_0 [Ohm]
  Constant : Constant  Value=ones(SysPara.p,1)  VectorParams1D=off
  Divide : Product  Inputs=*/
  Divide1 : Product  Inputs=*/
  Divide2 : Product  Inputs=*/
  Math Function : Math  Operator=reciprocal  SaturateOnIntegerOverflow=on
  Matrix Sum : Sum  Inputs=+  CollapseMode=Specified dimension
  Matrix Sum1 : Sum  Inputs=+  CollapseMode=Specified dimension
  Matrix Sum2 : Sum  Inputs=+  CollapseMode=Specified dimension
  Product : Product  Multiplication=Matrix(*)
  Subtract : Sum  Inputs=+-
  U_Cell [V] : Outport
  I_Cell [A] : Outport  Port=2
  U_R [V] : Outport  Port=3
  wires:
  Divide/1 -> Matrix Sum1/1
  I_Pack [A]/1 -> Add/2
  Matrix Sum1/1 -> Add/3
  Math Function/1 -> Matrix Sum2/1
  Add/1 -> Divide1/1
  Matrix Sum2/1 -> Divide1/2
  Divide1/1 -> Product/2
  Constant/1 -> Product/1
  Product/1 -> Subtract/1, U_Cell [V]/1  "U_cell [V]"
  Subtract/1 -> Divide2/1, U_R [V]/1  "U_R [V]"
  Divide2/1 -> I_Cell [A]/1  "I_cell [A]"
  Bus Selector1/1 -> Divide/2, Divide2/2, Math Function/1  "<R_0 [Ohm]>"
  Matrix Sum/1 -> Add/1
  I_Balancing_in [A]/1 -> Matrix Sum/1
  U_Potential [V]/1 -> Divide/1, Subtract/2
  BatPara/1 -> Bus Selector1/1

== system sim_BTMS/Battery system simulation/Electrical Submodel/Voltage of battery system ==
  note: Determination of the terminal voltage of the battery pack:
      | 1. Interconnection mechanism of the cells: Cells are first connected in parallel to a group à parallel cell groups are then connected in series
      | 2. Terminal voltage of a parallel cell network corresponds to the individual terminal voltages of the cells in this network.
      | 3. The total voltage of a serial circuit is the sum of its individual voltages.
      | 4. U_Pack (terminal voltage of the battery pack) = sum of the terminal voltages of the serially connected parallel cell composites
  U_Cells [V] : Inport
  Matrix Sum : Sum  Inputs=+
  Multiport Selector : dspindex/Multiport Selector  rowsOrCols=Rows  idxCellArray=1  idxErrMode=Clip Index
  U_Pack [V] : Outport
  wires:
  Matrix Sum/1 -> U_Pack [V]/1  "U_Pack [V]"
  U_Cells [V]/1 -> Multiport Selector/1
  Multiport Selector/1 -> Matrix Sum/1

== system sim_BTMS/Battery system simulation/Electrical Submodel/dt ==
  Clock : Clock
  Subtract : Sum  Inputs=+-
  Unit Delay : UnitDelay  SampleTime=-1
  dt [s] : Outport
  wires:
  Unit Delay/1 -> Subtract/2
  Clock/1 -> Unit Delay/1, Subtract/1
  Subtract/1 -> dt [s]/1
